simulink model "generic_IVS"  (R2024a)
settings: Solver=FixedStepDiscrete  StartTime=0.0  StopTime=inf  FixedStep=0.001  RelTol=1e-3  EnableMultiTasking=on
undefined symbols (not defined in the file): carLengthObs, dir, ego_Accel, ego_Speed, ego_X, ego_Y, ego_YAW, goalPosTol, goalYawTol, init_CurrentLaneInfo, init_DrivingMissionInfo, init_EgoVehicle, init_HybridAStarParam, init_MapData, init_ParkingMIssionInfo, is_Optimal_Path, isPathFound, LAD, lane_Coeff, lane_Idx, lane_waypoints, lane_waypoints_Length, lookAheadDistance, maxIter, missionState, obsRadius, parking_clear, parkingDestinationPos_X, parkingDestinationPos_Y, parkingDestinationYaw, parkingMapBoundary_X_Max, parkingMapBoundary_X_Min, parkingMapBoundary_Y_Max, parkingMapBoundary_Y_Min, parkingStartPos_X, parkingStartPos_Y, R_min, reversePenalty, Route1, route1_waypoint, Route2, route2_waypoint, Route3, route3_waypoint, Route_Parking, route_parking_waypoint, steerSet, stepSize, tollgateLaneNumber, vehicleRadius, velReference, xyResolution, y_LAD, y_lookAheadDistance, yawResolution, yawWeight
libraries: CarMaker4SL x53, simulink x1
(part 4 of 4)

== matlab function generic_IVS/CarMaker/Subsystem/Final Project/Scenario 1/Subsystem13/Optimal Trajectory Planner ==
  settings: sampleTime=0.05
  data: MapData_Info input; ego_status input; global_waypoints output size=[50 2]; otherVehicles input; driving_mission_info_in input Bus: busDrivingMissionInfo; driving_mission_info_out output Bus: busDrivingMissionInfo
function [global_waypoints, driving_mission_info_out]  = optimal_trajectory_planner(MapData_Info, ego_status, otherVehicles, driving_mission_info_in)
    [global_waypoints, driving_mission_info_out]  = optimal_trajectory_planner_m(MapData_Info, ego_status, otherVehicles, driving_mission_info_in);
end

== matlab function generic_IVS/CarMaker/Subsystem/Final Project/Scenario 1/Subsystem13/get_adj_obstacles_info ==
  settings: sampleTime=0.05
  data: ego_status input; obstacles_info input [3..10]; adj output size=[8 10]; driving_mission_info input
function adj = get_adj_obstacles_info(ego_status, obstacles_info, driving_mission_info)
    adj = get_adj_obstacles_info_m(ego_status, obstacles_info, driving_mission_info);
end

== matlab function generic_IVS/CarMaker/Subsystem/Final Project/Scenario 1/Set Velocity Reference ==
  settings: updateMethod=DISCRETE  sampleTime=0.05
  data: ego_status input Bus: busEgoVehicle; driving_mission_info_out output Bus: busDrivingMissionInfo; driving_mission_info_in input
function driving_mission_info_out = set_velocity_ref(ego_status, driving_mission_info_in)
    driving_mission_info_out = set_velocity_ref_m(ego_status, driving_mission_info_in);
end

== matlab function generic_IVS/CarMaker/Subsystem/Final Project/Scenario 1/MATLAB Function ==
  data: parking_mission_info input Bus: busParkingMissionInfo; path output size=[20000 4]; obstacles input; param input Bus: busHybridAStarParam
function path = hybridAstar_planner(parking_mission_info, obstacles, param)
    path = hybridAstar_planner_m(parking_mission_info, obstacles, param);
end

== matlab function generic_IVS/CarMaker/Subsystem/Final Project/Scenario 1/Global Waypoints To Local Transfomer ==
  settings: sampleTime=0.05
  data: mission_state input; parking_mission_info_in input Bus: busParkingMissionInfo; parking_mission_info_out output Bus: busParkingMissionInfo; waypoints input; ego_status input Bus: busEgoVehicle
function parking_mission_info_out  = global_to_local_path_manager(mission_state, parking_mission_info_in, waypoints, ego_status)
    parking_mission_info_out  = global_to_local_path_manager_m(mission_state, parking_mission_info_in, waypoints, ego_status);
end

== stateflow chart generic_IVS/CarMaker/Subsystem/Final Project/Scenario 1/Subsystem7/Chart3 ==
  state driving
    mission=1;
  state tollgate
    mission=2;
  state parking_entry
    mission=3;
  state parking
    mission=4;
  (default) -> driving
  driving -> tollgate [order 1] : [flag_2==1]
  tollgate -> driving : [flag_2==0]
  driving -> parking_entry [order 2] : [flag_3==1]
  parking_entry -> parking : [flag_4==1]
  data: flag_2 input; flag_3 input; mission output; flag_4 input

== matlab function generic_IVS/CarMaker/Subsystem/Final Project/Scenario 1/Subsystem6/MATLAB Function9 ==
  data: ego_status input; tollgate_pass_mode output
function tollgate_pass_mode = check_tollgate(ego_status)
% CHECK_TOLLGATE_ZONE: 에고 차량이 톨게이트 영역 내에 있는지 확인하여 플래그를 반환합니다.
%
% 입력:
%   ego_global_x: 에고 차량의 현재 글로벌 X 좌표 (float)
%   ego_global_y: 에고 차량의 현재 글로벌 Y 좌표 (float)


% 출력:
%   tollgate_pass_mode: 0 (영역 밖) 또는 1 (영역 내) (int)

    % 1. 톨게이트 영역 경계 정의
    min_x = -190;
    max_x = -90;
    min_y = -165;
    max_y = -86;
    
    ego_global_x = ego_status.ego_X;
    ego_global_y = ego_status.ego_Y;

    % 2. 플래그 설정 로직
    if (ego_global_x >= min_x && ego_global_x <= max_x) && ...
       (ego_global_y >= min_y && ego_global_y <= max_y)
        % 에고 차량이 영역 내에 있는지 확인
        tollgate_pass_mode = 1;
    else
        % 그렇지 않을 경우 (영역 밖)
        tollgate_pass_mode = 0;
    end
    
    %
end

== matlab function generic_IVS/CarMaker/Subsystem/Final Project/Scenario 1/Subsystem6/MATLAB Function10 ==
  data: ego_status input; parking_entry_mode output; IS_FRONT input
function parking_entry_mode = check_parking_entry(ego_status, IS_FRONT)
    % Simulink MATLAB Function 블록용 주차 진입 플래그 로직 (수정됨)
    
    % 영구 변수(Persistent Variables) 선언
    persistent parking_entry_flag Pass_Count In_Boundary_Prev TARGET_PASS_COUNT IsInitialized
    parking_entry_mode = uint8(0);

    Ego_Global_X = ego_status.ego_X;
    Ego_Global_Y = ego_status.ego_Y;
    % BOUNDARY 변수 정의 (시뮬레이션 환경에 맞게 조정 필요)
    BOUND_X_MIN = -108;
    BOUND_X_MAX = -95;
    BOUND_Y_MIN = -3;
    BOUND_Y_MAX = 17;
    
    % X_MAX = -95;
    % X_MIN = -108;
    % Y_MIN = 3;
    % Y_MAX = 17;
    
    % --- 1. 초기화 (시뮬레이션 시작 시 단 한 번 실행) ---
    if isempty(IsInitialized)
        
        % A. IS_FRONT 값에 기반하여 Target_Pass_Count 설정
        if IS_FRONT == 1
            % 앞 시작: 1번째 진입 시 플래그 활성화
            TARGET_PASS_COUNT = uint8(1); 
        else
            % 뒤 시작: 2번째 진입 시 플래그 활성화
            TARGET_PASS_COUNT = uint8(2);
        end
    
        % 초기 상태 설정 (타입 캐스팅 적용)
        parking_entry_flag = uint8(0);
        Pass_Count = uint8(0);         
        In_Boundary_Prev = false; 
        IsInitialized = true;
    end
    
    % --- 2. 실시간 업데이트 (매 스텝마다 실행) ---
    
    % 1. 이미 플래그가 1이면 더 이상 계산할 필요 없음
    if parking_entry_flag == 1
        parking_entry_flag = uint8(parking_entry_flag);
        return;
    end
    
    % 2. 현재 바운더리 상태 확인
    In_Boundary_Curr = (Ego_Global_X >= BOUND_X_MIN && Ego_Global_X <= BOUND_X_MAX && ...
                        Ego_Global_Y >= BOUND_Y_MIN && Ego_Global_Y <= BOUND_Y_MAX);
    
    % 3. 통과 횟수 업데이트 (밖 -> 안 진입 감지)
    if In_Boundary_Curr && ~In_Boundary_Prev
        Pass_Count = Pass_Count + uint8(1);
    end
    
    % 4. 플래그 활성화 조건 확인
    % Pass_Count가 목표 횟수와 같아지는 순간 플래그 활성화
    if Pass_Count == TARGET_PASS_COUNT
        parking_entry_flag = uint8(1);
    end
    
    % 5. 다음 스텝을 위한 상태 저장
    In_Boundary_Prev = In_Boundary_Curr;
    
    parking_entry_mode = uint8(parking_entry_flag); 

end

== matlab function generic_IVS/CarMaker/Subsystem/Final Project/Scenario 1/Subsystem6/MATLAB Function11 ==
  data: ego_status input; parking_mode output
function parking_mode = check_parking_zone(ego_status)


% 입력:
%   ego_global_x: 에고 차량의 현재 글로벌 X 좌표 (float)
%   ego_global_y: 에고 차량의 현재 글로벌 Y 좌표 (float)
%   tollgate_zone_x_limits: 톨게이트 영역의 X축 경계 [min_x, max_x]
%   tollgate_zone_y_limits: 톨게이트 영역의 Y축 경계 [min_y, max_y]
%
% 출력:
%   주차장 모드 0 (영역 밖) 또는 1 (영역 내) (int)
    
    parking_mode = 0;

    ego_global_X = ego_status.ego_X;
    ego_global_Y = ego_status.ego_Y;
    % 1. 주차장 영역 -> 여기로 들어오면 parking
    min_x = -2.5;
    max_x = 5.5;
    min_y = -38.5;
    max_y = -25.0;

    % 2. 플래그 설정 로직
    if (ego_global_X >= min_x && ego_global_X <= max_x) && ...
       (ego_global_Y >= min_y && ego_global_Y <= max_y)
        
        parking_mode = 1;
    end
    
end

== matlab function generic_IVS/CarMaker/Subsystem/Final Project/Scenario 1/Subsystem11/Lateral Control/MATLAB Function8 ==
  settings: updateMethod=DISCRETE  sampleTime=0.01
  data: parking_mission_info input Bus: busParkingMissionInfo; delta output; ego_status input
function delta  = lateral_PP_controller_parking(parking_mission_info, ego_status)
    delta  = lateral_PP_controller_parking_m(parking_mission_info, ego_status);
end

== stateflow chart generic_IVS/CarMaker/Subsystem/Day3/Chart ==
  (default) -> (junction 1)
  (junction 1) -> (junction 3) [order 1] : [i<99]
      | {i = i + 1;}
  (junction 1) -> (junction 7) [order 2] : {i=0;}
  (junction 3) -> (junction 5)
  (junction 5) -> (junction 7)
  (junction 7) -> (junction 10)
  (junction 10) -> (junction 12) [order 1] : [rem(i,50) == 0]
      | {do_Logic;}
  (junction 10) -> (junction 18) [order 2]
  (junction 12) -> (junction 16)
  (junction 16) -> (junction 18)
  (junction 18) -> (junction 21)
  data: i local =0
  events: do_Logic output FUNCTION_CALL_EVENT
